simulink model "FirstPrincChambOnly_Testing"  (R2025b)
settings: Solver=VariableStepAuto  StartTime=0.0  StopTime=10.0  RelTol=1e-3
undefined symbols (not defined in the file): A_t, cstar_matr, k_d_chamb, mdot_f_nom_cstar_match, mdot_ox_nom_cstar_match, OF_vec, P_amb, Pc_vec, psi_to_Pa, sonvel_matr, V_c
settings Model: Creator=gruby  LastModifiedBy=gruby

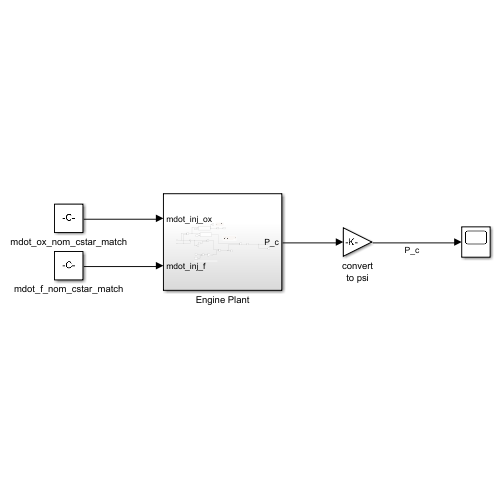
[thumbnail: Simulink's stored preview of the top-level diagram]
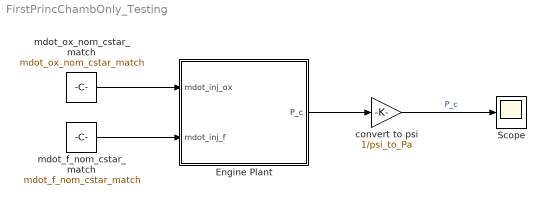
== system FirstPrincChambOnly_Testing ==
  Engine Plant : Subsystem
  Scope : Scope
      settings: ActiveDisplayYMinimum=349.25591542161266  ActiveDisplayYMaximum=350.136792302115
  convert to psi : Gain  Gain=1/psi_to_Pa
  mdot_f_nom_cstar_match : Constant  Value=mdot_f_nom_cstar_match
  mdot_ox_nom_cstar_match : Constant  Value=mdot_ox_nom_cstar_match
  wires:
  Engine Plant/1(P_c) -> convert to psi/1
  convert to psi/1 -> Scope/1  "P_c"
  mdot_f_nom_cstar_match/1 -> Engine Plant/2(mdot_inj_f)
  mdot_ox_nom_cstar_match/1 -> Engine Plant/1(mdot_inj_ox)

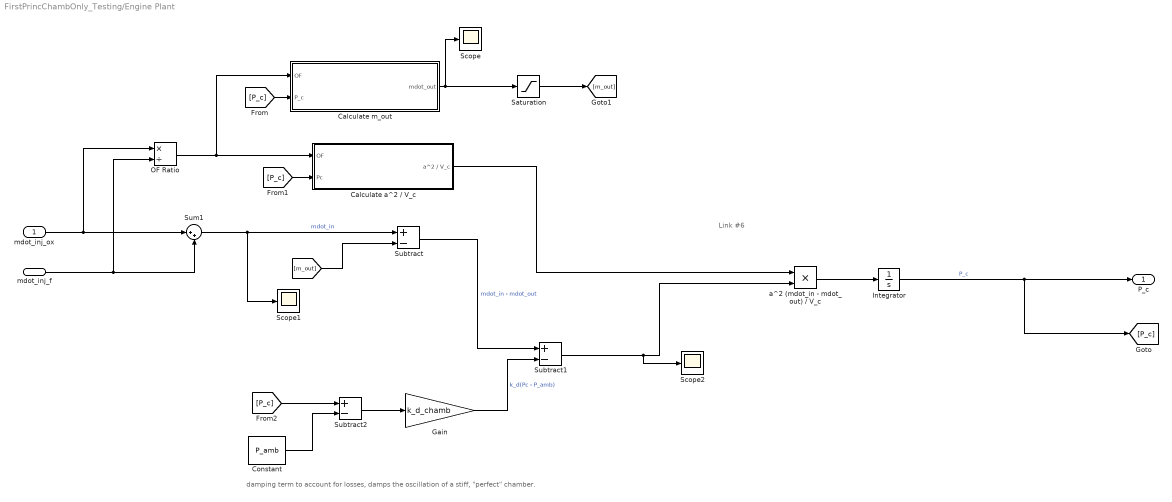
== system FirstPrincChambOnly_Testing/Engine Plant ==
  note: damping term to account for losses, damps the oscillation of a stiff, "perfect" chamber.
  note: Link #6
  mdot_inj_ox : Inport
  mdot_inj_f : Inport  Port=2
  Calculate a^2 / V_c : Subsystem
  Calculate m_out : Subsystem
  Constant : Constant  Value=P_amb
  Gain : Gain  Gain=k_d_chamb
  Integrator : Integrator  InitialCondition=P_amb
  OF Ratio : Product  Inputs=*/
  Saturation : Saturate  UpperLimit=+Inf  LowerLimit=1e-8
  Scope : Scope
      settings: ActiveDisplayYMinimum=-0.1596972694404093  ActiveDisplayYMaximum=0.5680503720193445  DataLoggingVariableName=ScopeData16
  Scope1 : Scope
      settings: ActiveDisplayYMinimum=-1  ActiveDisplayYMaximum=1  DataLoggingVariableName=ScopeData17
  Scope2 : Scope
      settings: ActiveDisplayYMinimum=-1  ActiveDisplayYMaximum=1
  Subtract : Sum  Inputs=+-
  Subtract1 : Sum  Inputs=+-
  Subtract2 : Sum  Inputs=+-
  Sum1 : Sum  Inputs=|++
  "a^2 (mdot_in - mdot_out) / V_c " : Product
  P_c : Outport
  wires:
  mdot_inj_f/1 -> OF Ratio/2, Sum1/2
  mdot_inj_ox/1 -> OF Ratio/1, Sum1/1
  Integrator/1 -> P_c/1, [P_c]  "P_c"
  OF Ratio/1 -> Calculate m_out/1(OF), Calculate a^2 / V_c/1(OF)
  "a^2 (mdot_in - mdot_out) / V_c "/1 -> Integrator/1
  [P_c] -> Calculate m_out/2(P_c)
  [P_c] -> Calculate a^2 / V_c/2(Pc)
  Calculate a^2 / V_c/1(a^2 / V_c) -> "a^2 (mdot_in - mdot_out) / V_c "/1
  Calculate m_out/1(mdot_out) -> Scope/1, Saturation/1
  [m_out] -> Subtract/2
  Sum1/1 -> Scope1/1, Subtract/1  "mdot_in"
  Subtract/1 -> Subtract1/1  "mdot_in - mdot_out"
  Saturation/1 -> [m_out]
  [P_c] -> Subtract2/1
  Constant/1 -> Subtract2/2
  Subtract2/1 -> Gain/1
  Gain/1 -> Subtract1/2  "k_d(Pc - P_amb)"
  Subtract1/1 -> Scope2/1, "a^2 (mdot_in - mdot_out) / V_c "/2

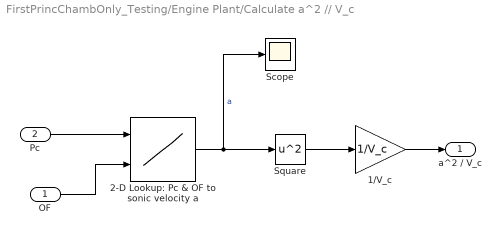
== system FirstPrincChambOnly_Testing/Engine Plant/Calculate a^2 // V_c ==
  OF : Inport
  Pc : Inport  Port=2
  1/V_c : Gain  Gain=1/V_c
  2-D Lookup: Pc & OF to sonic velocity a : Lookup_n-D  BreakpointsForDimension1=Pc_vec  BreakpointsForDimension2=OF_vec  Table=sonvel_matr  ExtrapMethod=Clip  UseLastTableValue=on  InternalRulePriority=Speed  RndMeth=Simplest
      settings: InputPortMap=u0,u1
  Scope : Scope
      settings: ActiveDisplayYMinimum=-1  ActiveDisplayYMaximum=1  DataLoggingVariableName=ScopeData15
  Square : Math  Operator=square
  a^2 / V_c : Outport
  wires:
  2-D Lookup: Pc & OF to sonic velocity a/1 -> Scope/1, Square/1  "a"
  Square/1 -> 1/V_c/1
  1/V_c/1 -> a^2 / V_c/1
  OF/1 -> 2-D Lookup: Pc & OF to sonic velocity a/2
  Pc/1 -> 2-D Lookup: Pc & OF to sonic velocity a/1

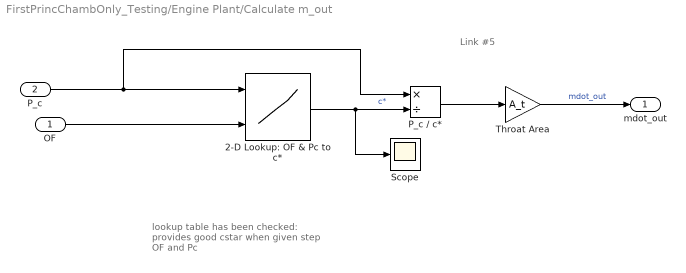
== system FirstPrincChambOnly_Testing/Engine Plant/Calculate m_out ==
  note: lookup table has been checked: provides good cstar when given step OF and Pc
  note: Link #5
  OF : Inport
  P_c : Inport  Port=2
  2-D Lookup: OF & Pc to c* : Lookup_n-D  BreakpointsForDimension1=Pc_vec  BreakpointsForDimension2=OF_vec  Table=cstar_matr  ExtrapMethod=Clip  UseLastTableValue=on  InternalRulePriority=Speed  RndMeth=Simplest
      settings: InputPortMap=u0,u1
  P_c / c* : Product  Inputs=*/
  Scope : Scope
      settings: ActiveDisplayYMinimum=-1  ActiveDisplayYMaximum=1  DataLoggingVariableName=ScopeData24
  Throat Area : Gain  Gain=A_t
  mdot_out : Outport
  wires:
  2-D Lookup: OF & Pc to c*/1 -> Scope/1, P_c / c*/2  "c*"
  P_c / c*/1 -> Throat Area/1
  OF/1 -> 2-D Lookup: OF & Pc to c*/2
  Throat Area/1 -> mdot_out/1  "mdot_out"
  P_c/1 -> P_c / c*/1, 2-D Lookup: OF & Pc to c*/1
